simulink model "lab_5_task_1"  (R2023b)
settings: Solver=VariableStepAuto  StartTime=0.0  StopTime=10.0  RelTol=1e-3
settings Model: Creator=f_mes  LastModifiedBy=f_mes

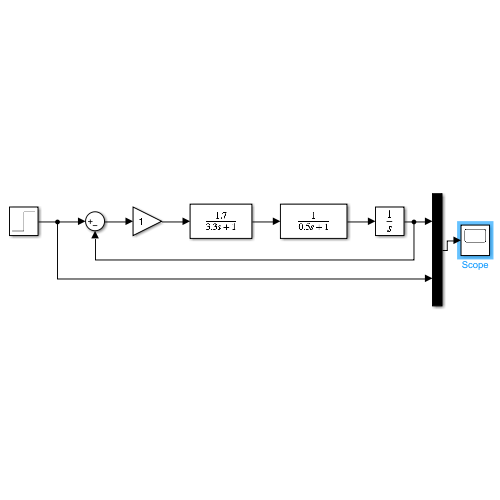
[thumbnail: Simulink's stored preview of the top-level diagram]
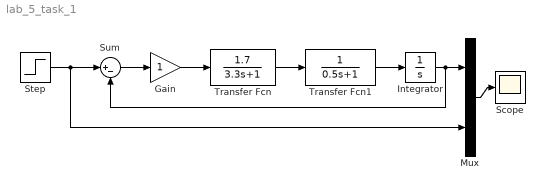
== system lab_5_task_1 ==
  Gain : Gain
  Integrator : Integrator
  Mux : Mux  Inputs=2
  Scope : Scope
  Step : Step  Time=0  SampleTime=0
  Sum : Sum  Inputs=|+-
  Transfer Fcn : TransferFcn  Numerator=[1.7]  Denominator=[3.3, 1]  ParameterTunability=Unconstrained
  Transfer Fcn1 : TransferFcn  Denominator=[0.5, 1]
  wires:
  Sum/1 -> Gain/1
  Gain/1 -> Transfer Fcn/1
  Transfer Fcn/1 -> Transfer Fcn1/1
  Transfer Fcn1/1 -> Integrator/1
  Mux/1 -> Scope/1
  Integrator/1 -> Sum/2, Mux/1
  Step/1 -> Mux/2, Sum/1
